simulink model "pm_a"  (R2023a)
settings: Solver=FixedStepAuto  StartTime=0.0  StopTime=0.1  FixedStep=0.0001  RelTol=1e-3
settings Model: Creator=pasha  LastModifiedBy=tanov

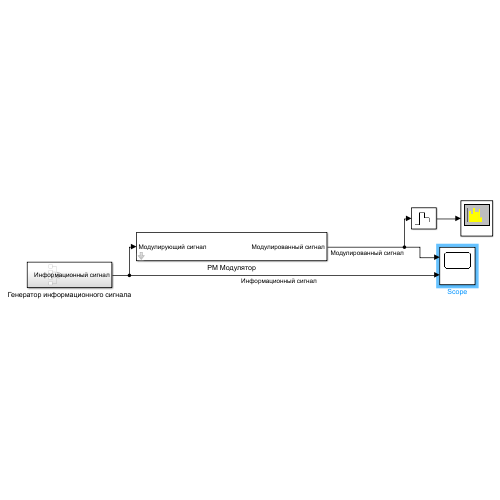
[thumbnail: Simulink's stored preview of the top-level diagram]
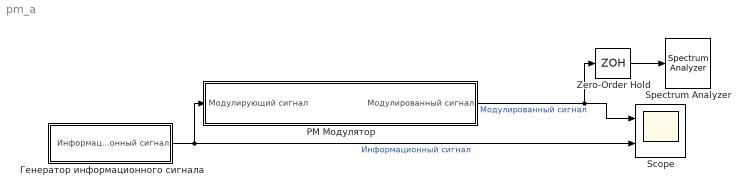
== system pm_a ==
  PM Модулятор : Subsystem  mask{f_c=300, m=0.01}
      mask prompts: f_c "Частота несущей"; m "Девиация Фазы"
  Scope : Scope  NumInputPorts=2
  Spectrum Analyzer : SpectrumAnalyzer  WindowPosition=[1.000000,49.000000,1600.000000,930.000000,]  ScopeFrameLocation=window  YLimits=[-57.89747678,31.43634505]
  Zero-Order Hold : ZeroOrderHold  SampleTime=1e-3
  Генератор информационного сигнала : Subsystem
  wires:
  Генератор информационного сигнала/1(Информационный сигнал) -> PM Модулятор/1(Модулирующий сигнал), Scope/2  "Информационный сигнал"
  Zero-Order Hold/1 -> Spectrum Analyzer/1
  PM Модулятор/1(Модулированный сигнал) -> Scope/1, Zero-Order Hold/1  "Модулированный сигнал"

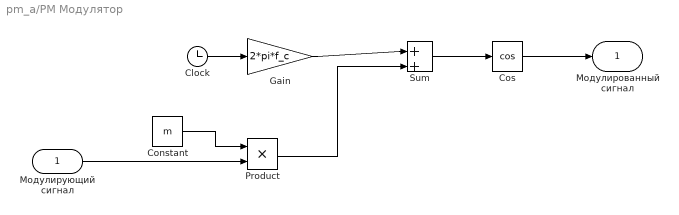
== system pm_a/PM Модулятор ==
  Модулирующий сигнал : Inport
  Clock : Clock
  Constant : Constant  Value=m
  Cos : Trigonometry  Operator=cos
  Gain : Gain  Gain=2*pi*f_c
  Product : Product
  Sum : Sum  Inputs=|++
  Модулированный сигнал : Outport
  wires:
  Модулирующий сигнал/1 -> Product/2
  Constant/1 -> Product/1
  Clock/1 -> Gain/1
  Product/1 -> Sum/2
  Sum/1 -> Cos/1
  Cos/1 -> Модулированный сигнал/1
  Gain/1 -> Sum/1

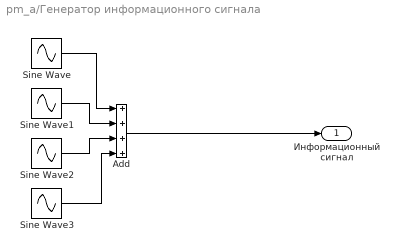
== system pm_a/Генератор информационного сигнала ==
  Add : Sum  Inputs=++++
  Sine Wave : Sin  Frequency=2*pi*40  SampleTime=0
  Sine Wave1 : Sin  Frequency=2*pi*60  SampleTime=0
  Sine Wave2 : Sin  Frequency=2*pi*80  SampleTime=0
  Sine Wave3 : Sin  Frequency=2*pi*100  SampleTime=0
  Информационный сигнал : Outport
  wires:
  Sine Wave/1 -> Add/1
  Sine Wave3/1 -> Add/4
  Sine Wave1/1 -> Add/2
  Sine Wave2/1 -> Add/3
  Add/1 -> Информационный сигнал/1
